simulink model "Modelo_Tanque_Controlado_Malha_Fechada"  (R2023a)
settings: Solver=FixedStepAuto  StartTime=0.0  StopTime=5000  FixedStep=1e-3  RelTol=1e-3
libraries: simulink x1
settings Model: Creator=User  LastModifiedBy=dougl
settings DebuggingCC: UnconnectedInputMsg=warning  UnconnectedOutputMsg=warning  UnconnectedLineMsg=warning
settings ModelReferenceCC: EnableRefExpFcnMdlSchedulingChecks=on
settings RTWCC: DLArmComputeVersion=19.05

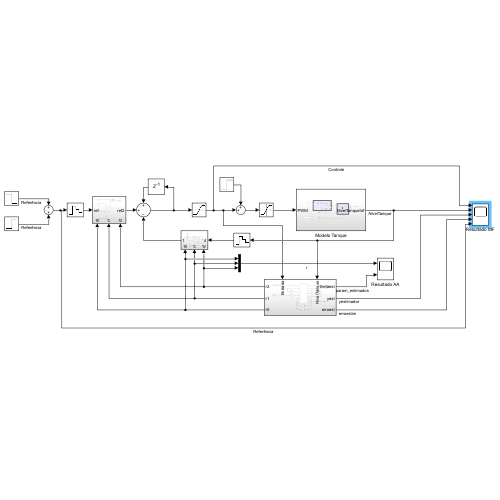
[thumbnail: Simulink's stored preview of the top-level diagram]
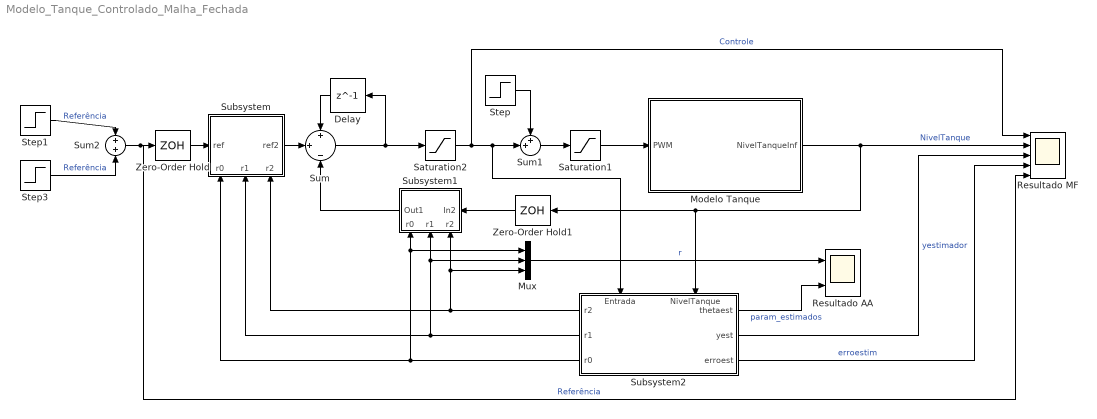
== system Modelo_Tanque_Controlado_Malha_Fechada ==
  Delay : Delay  DelayLength=1  SampleTime=10
  Modelo Tanque : Subsystem
  Mux : Mux  Inputs=3
  Resultado AA : Scope  NumInputPorts=2
  Resultado MF : Scope  NumInputPorts=5
  Saturation1 : Saturate  UpperLimit=1  LowerLimit=0
  Saturation2 : Saturate  UpperLimit=1  LowerLimit=0
  Step : Step  Time=3500  After=0.1  SampleTime=0
  Step1 : Step  Time=1500  Before=2  After=0.5  SampleTime=0
  Step3 : Step  Time=2500  After=0.5  SampleTime=0
  Subsystem : Subsystem
      settings: PortSchema="{\"entries\":[{\"content\":{\"sides\":[{\"content\":{\"connectorIds\":[\"In1\"]},\"type\":\"ConnectorPlacement.EquallySpacedRectSide\",\"uuid\":\"54959ef1-1612-4867-ba6b-dc765a8ddae4\"},{\"content\":{\"connectorIds\":[\"Out1\"],\"side\":\"RIGHT\"},\"type\":\"ConnectorPlacement.EquallySpacedRectSide\",\"uuid\":\"521d5a99-2882-44a0-898b-5bf67ff27f87\"},{\"content\":{\"connectorIds\":[],\"side\":\"TOP\"},\"type\":\"ConnectorPlacement.EquallySpacedRectSide\",\"uuid\":\"ae44589a-6dbf-4b55-9a6a-5a2b0c589258\"},{\"content\":{\"connectorIds\":[\"In2\",\"In3\",\"In4\"],\"side\":\"BOTTOM\"},\"type\":\"ConnectorPlacement.EquallySpacedRectSide\",\"uuid\":\"b8a51d85-951b-4d0a-aebc-145a9bace802\"}]},\"type\":\"ConnectorPlacement.EquallySpacedConnector\",\"uuid\":\"8bb11b5c-8b9f-451d-a3f4-37254325d24b\"}],\"packageUris\":[\"http://schema.mathworks.com/mf0/Connector/R2020b\"],\"version\":\"1.0\"}"
  Subsystem1 : Subsystem
      settings: PortSchema="{\"entries\":[{\"content\":{\"sides\":[{\"content\":{\"connectorIds\":[\"In1\",\"In2\",\"In3\"]},\"type\":\"ConnectorPlacement.EquallySpacedRectSide\",\"uuid\":\"54959ef1-1612-4867-ba6b-dc765a8ddae4\"},{\"content\":{\"connectorIds\":[],\"side\":\"RIGHT\"},\"type\":\"ConnectorPlacement.EquallySpacedRectSide\",\"uuid\":\"521d5a99-2882-44a0-898b-5bf67ff27f87\"},{\"content\":{\"connectorIds\":[\"Out1\"],\"side\":\"TOP\"},\"type\":\"ConnectorPlacement.EquallySpacedRectSide\",\"uuid\":\"ae44589a-6dbf-4b55-9a6a-5a2b0c589258\"},{\"content\":{\"connectorIds\":[\"In4\"],\"side\":\"BOTTOM\"},\"type\":\"ConnectorPlacement.EquallySpacedRectSide\",\"uuid\":\"8dea5e0f-1f05-4852-a966-a18b3b0c3dd8\"}]},\"type\":\"ConnectorPlacement.EquallySpacedConnector\",\"uuid\":\"8bb11b5c-8b9f-451d-a3f4-37254325d24b\"}],\"packageUris\":[\"http://schema.mathworks.com/mf0/Connector/R2020b\"],\"version\":\"1.0\"}"
  Subsystem2 : Subsystem
      settings: PortSchema="{\"entries\":[{\"content\":{\"sides\":[{\"content\":{\"connectorIds\":[\"In1\",\"In2\"]},\"type\":\"ConnectorPlacement.EquallySpacedRectSide\",\"uuid\":\"af01629c-d48c-45bc-b24d-07cc3b6a4066\"},{\"content\":{\"connectorIds\":[],\"side\":\"RIGHT\"},\"type\":\"ConnectorPlacement.EquallySpacedRectSide\",\"uuid\":\"5cb35106-4220-4a2a-b18c-340f924146f2\"},{\"content\":{\"connectorIds\":[\"Out4\",\"Out5\",\"Out6\"],\"side\":\"TOP\"},\"type\":\"ConnectorPlacement.EquallySpacedRectSide\",\"uuid\":\"758aa1a9-d53b-4379-b222-a0bce0ffcca4\"},{\"content\":{\"connectorIds\":[\"Out1\",\"Out2\",\"Out3\"],\"side\":\"BOTTOM\"},\"type\":\"ConnectorPlacement.EquallySpacedRectSide\",\"uuid\":\"8bde2633-f277-4a21-8538-53f5a0361e49\"}]},\"type\":\"ConnectorPlacement.EquallySpacedConnector\",\"uuid\":\"98ec68b8-fe21-420e-85fb-090df0d803e4\"}],\"packageUris\":[\"http://schema.mathworks.com/mf0/Connector/R2020b\"],\"version\":\"1.0\"}"
  Sum : Sum  Inputs=+|+|-
  Sum1 : Sum  Inputs=++|
  Sum2 : Sum  Inputs=+|+
  Zero-Order Hold : ZeroOrderHold  SampleTime=10
  Zero-Order Hold1 : ZeroOrderHold  SampleTime=10
  wires:
  Modelo Tanque/1(NivelTanqueInf) -> Subsystem2/2(NivelTanque), Zero-Order Hold1/1, Resultado MF/2  "NivelTanque"
  Delay/1 -> Sum/1
  Sum/1 -> Saturation2/1, Delay/1
  Zero-Order Hold/1 -> Subsystem/1(ref)
  Subsystem/1(ref2) -> Sum/2
  Zero-Order Hold1/1 -> Subsystem1/4(In2)
  Subsystem1/1(Out1) -> Sum/3
  Subsystem2/6(r0) -> Mux/1, Subsystem1/1(r0), Subsystem/2(r0)
  Subsystem2/5(r1) -> Subsystem/3(r1), Mux/2, Subsystem1/2(r1)
  Subsystem2/4(r2) -> Mux/3, Subsystem1/3(r2), Subsystem/4(r2)
  Subsystem2/2(yest) -> Resultado MF/3  "yestimador"
  Subsystem2/1(thetaest) -> Resultado AA/2  "param_estimados"
  Subsystem2/3(erroest) -> Resultado MF/4  "erroestim"
  Saturation1/1 -> Modelo Tanque/1(PWM)
  Saturation2/1 -> Resultado MF/1, Sum1/2, Subsystem2/1(Entrada)  "Controle"
  Step1/1 -> Sum2/1  "Referência"
  Step3/1 -> Sum2/2  "Referência"
  Sum2/1 -> Resultado MF/5, Zero-Order Hold/1  "Referência"
  Mux/1 -> Resultado AA/1  "r"
  Sum1/1 -> Saturation1/1
  Step/1 -> Sum1/1

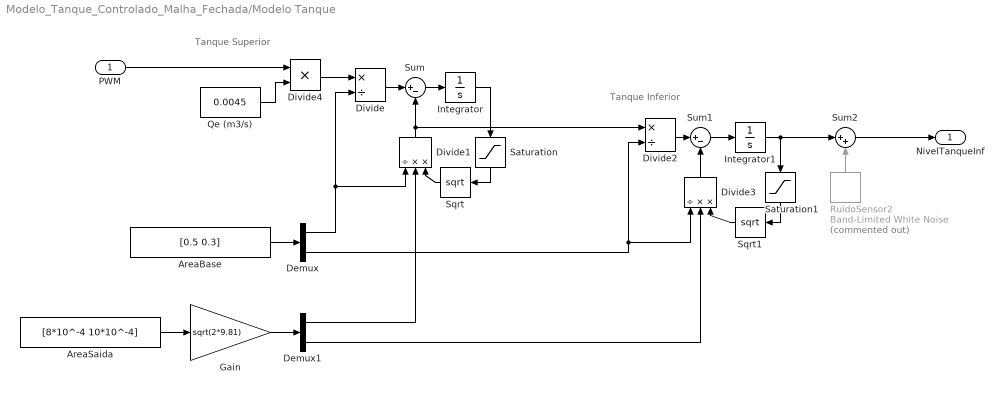
== system Modelo_Tanque_Controlado_Malha_Fechada/Modelo Tanque ==
  note: Tanque Inferior
  note: Tanque Superior
  PWM : Inport
  AreaBase : Constant  Value=[0.5 0.3]
  AreaSaida : Constant  Value=[8*10^-4 10*10^-4]
  Demux : Demux  Outputs=2
  Demux1 : Demux  Outputs=2
  Divide : Product  Inputs=*/
  Divide1 : Product  Inputs=/**
  Divide2 : Product  Inputs=*/
  Divide3 : Product  Inputs=/**
  Divide4 : Product  Inputs=**
  Gain : Gain  Gain=sqrt(2*9.81)
  Integrator : Integrator
  Integrator1 : Integrator
  Qe (m3/s) : Constant  Value=0.0045
  RuidoSensor2 : simulink/Sources/Band-Limited White Noise  Commented=on  Cov=[0.00001]  Ts=1  seed=[23341]
  Saturation : Saturate  UpperLimit=inf  LowerLimit=0
  Saturation1 : Saturate  UpperLimit=inf  LowerLimit=0
  Sqrt : Sqrt
  Sqrt1 : Sqrt
  Sum : Sum  Inputs=|+-
  Sum1 : Sum  Inputs=|+-
  Sum2 : Sum  Inputs=|++
  NivelTanqueInf : Outport
  wires:
  AreaSaida/1 -> Gain/1
  AreaBase/1 -> Demux/1
  Gain/1 -> Demux1/1
  Integrator/1 -> Saturation/1
  Demux/1 -> Divide/2, Divide1/1
  Divide/1 -> Sum/1
  Sum/1 -> Integrator/1
  Demux1/1 -> Divide1/2
  Sqrt/1 -> Divide1/3
  Integrator1/1 -> Saturation1/1, Sum2/1
  Demux1/2 -> Divide3/2
  Sqrt1/1 -> Divide3/3
  Divide3/1 -> Sum1/2
  Demux/2 -> Divide3/1, Divide2/2
  Sum1/1 -> Integrator1/1
  Divide2/1 -> Sum1/1
  Sum2/1 -> NivelTanqueInf/1
  RuidoSensor2/1 -> Sum2/2
  Divide1/1 -> Divide2/1, Sum/2
  Saturation/1 -> Sqrt/1
  Saturation1/1 -> Sqrt1/1
  Divide4/1 -> Divide/1
  Qe (m3/s)/1 -> Divide4/2
  PWM/1 -> Divide4/1

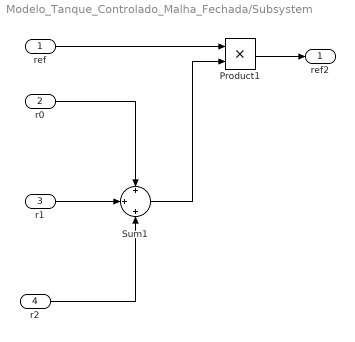
== system Modelo_Tanque_Controlado_Malha_Fechada/Subsystem ==
  ref : Inport
  r0 : Inport  Port=2
  r1 : Inport  Port=3
  r2 : Inport  Port=4
  Product1 : Product
  Sum1 : Sum  Inputs=+|+|+
  ref2 : Outport
  wires:
  ref/1 -> Product1/1
  Product1/1 -> ref2/1
  r0/1 -> Sum1/1
  r1/1 -> Sum1/2
  r2/1 -> Sum1/3
  Sum1/1 -> Product1/2

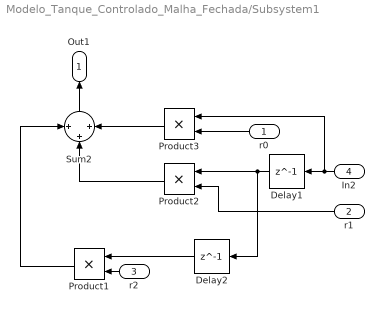
== system Modelo_Tanque_Controlado_Malha_Fechada/Subsystem1 ==
  r0 : Inport
  r1 : Inport  Port=2
  r2 : Inport  Port=3
  In2 : Inport  Port=4
  Delay1 : Delay  DelayLength=1  SampleTime=10
  Delay2 : Delay  DelayLength=1  SampleTime=10
  Product1 : Product
  Product2 : Product
  Product3 : Product
  Sum2 : Sum  Inputs=+|+|+
  Out1 : Outport
  wires:
  In2/1 -> Delay1/1, Product3/1
  Product3/1 -> Sum2/3
  Product2/1 -> Sum2/2
  r1/1 -> Product2/2
  Delay1/1 -> Product2/1, Delay2/1
  r0/1 -> Product3/2
  Sum2/1 -> Out1/1
  Delay2/1 -> Product1/1
  Product1/1 -> Sum2/1
  r2/1 -> Product1/2

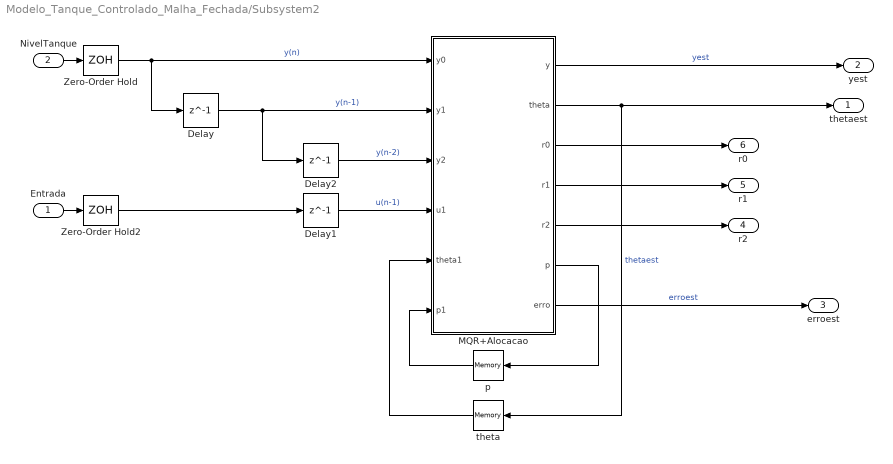
== system Modelo_Tanque_Controlado_Malha_Fechada/Subsystem2 ==
  Entrada : Inport
  NivelTanque : Inport  Port=2
  Delay : Delay  DelayLength=1  InitialCondition=0  SampleTime=10
  Delay1 : Delay  DelayLength=1  InitialCondition=0  SampleTime=10
  Delay2 : Delay  DelayLength=1  InitialCondition=0  SampleTime=10
  MQR+Alocacao : MATLAB Function  TreatAsAtomicUnit=on
  Zero-Order Hold : ZeroOrderHold  SampleTime=10
  Zero-Order Hold2 : ZeroOrderHold  SampleTime=10
  p : Memory  InitialCondition=100*eye(3)  InheritSampleTime=on
  theta : Memory  InitialCondition=[0; 0; 1]  InheritSampleTime=on
  thetaest : Outport
  yest : Outport  Port=2
  erroest : Outport  Port=3
  r2 : Outport  Port=4
  r1 : Outport  Port=5
  r0 : Outport  Port=6
  wires:
  Delay/1 -> MQR+Alocacao/2(y1), Delay2/1  "y(n-1)"
  MQR+Alocacao/6(p) -> p/1
  NivelTanque/1 -> Zero-Order Hold/1
  p/1 -> MQR+Alocacao/6(p1)
  Zero-Order Hold/1 -> Delay/1, MQR+Alocacao/1(y0)  "y(n)"
  Entrada/1 -> Zero-Order Hold2/1
  Delay2/1 -> MQR+Alocacao/3(y2)  "y(n-2)"
  MQR+Alocacao/2(theta) -> theta/1, thetaest/1  "thetaest"
  MQR+Alocacao/1(y) -> yest/1  "yest"
  theta/1 -> MQR+Alocacao/5(theta1)
  Delay1/1 -> MQR+Alocacao/4(u1)  "u(n-1)"
  Zero-Order Hold2/1 -> Delay1/1
  MQR+Alocacao/7(erro) -> erroest/1  "erroest"
  MQR+Alocacao/3(r0) -> r0/1
  MQR+Alocacao/4(r1) -> r1/1
  MQR+Alocacao/5(r2) -> r2/1

== matlab function Modelo_Tanque_Controlado_Malha_Fechada/Subsystem2/MQR+Alocacao ==
  data: y0 input; y1 input; y2 input; u1 input; theta1 input; p1 input; y output; theta output; r0 output; r1 output; r2 output; p output; erro output
function [y, theta, r0, r1, r2, p, erro] = fcn(y0, y1, y2, u1, theta1, p1)

lambda1 = 0.99;
lambda2 = 1;

lambda = lambda1/lambda2;

fi = [-y1;...
      -y2;...
       u1];

erro = y0-fi'*theta1;           % Calcula erro de estimação

k = p1*fi/(lambda+fi'*p1*fi);   % Atualiza vetor de ajuste do theta

theta=theta1+k*erro;            % Atualiza o theta

p=(p1-k*fi'*p1)/lambda1;        % Atualiza matriz de covariância

y = fi'*theta;                  % Calcula a saída a partir dos thetas estimados

a1 = theta(1);
a2 = theta(2);
b0 = theta(3);

polos = [1 -1.8097 0.8187];

r0 = (polos(2)+1-a1)/b0;
r1 = (polos(3)+a1-a2)/b0;
r2 = a2/b0;
